simulink model "model"  (R2024b)
settings: Solver=FixedStepAuto  StartTime=0.0  StopTime=159.6  FixedStep=Ts  RelTol=1e-3
values from neighbouring files (symbols this model uses):
  Ts = 0.25    [freq_domain.m]    (also in impulse_deconv.m = 0.4; impulse_resp_correlation.m; niel_week1to3.m = 0.4; script.m = 0.4)
settings Model: Creator=niel  LastModifiedBy=farahelsousy

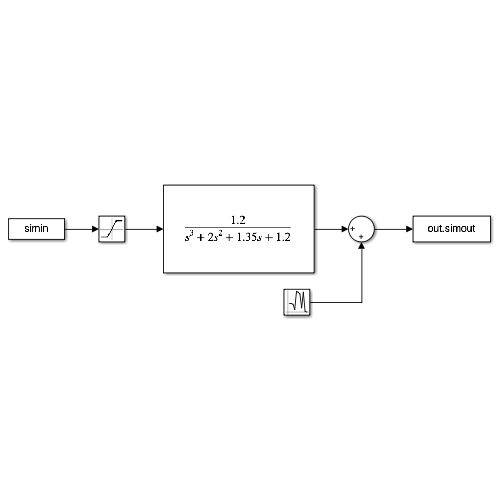
[thumbnail: Simulink's stored preview of the top-level diagram]
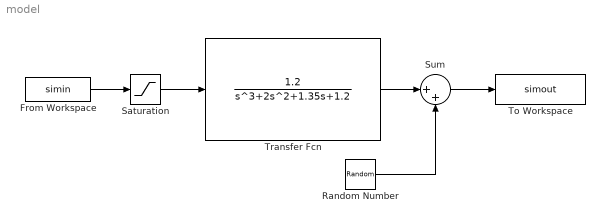
== system model ==
  From Workspace : FromWorkspace  VariableName=simin  SampleTime=Ts
  Random Number : RandomNumber  Variance=0.01  SampleTime=Ts
  Saturation : Saturate  UpperLimit=0.7  LowerLimit=-0.7
  Sum : Sum  Inputs=|++
  To Workspace : ToWorkspace  VariableName=simout  SaveFormat=Timeseries  SampleTime=Ts
  Transfer Fcn : TransferFcn  Numerator=[1.2]  Denominator=[1 2 1.35 1.2]  ParameterTunability=Optimized
  wires:
  Sum/1 -> To Workspace/1
  From Workspace/1 -> Saturation/1
  Saturation/1 -> Transfer Fcn/1
  Transfer Fcn/1 -> Sum/1
  Random Number/1 -> Sum/2
